simulink model "Diode"  (R2020a)
settings: Solver=VariableStepAuto  StartTime=0.0  StopTime=10.0  RelTol=1e-3
model workspace (MAT data in the model file):
  Eg = Simulink.Parameter
  Eg.Value = 1.23
  Eg.DataType = 'auto'
  Eg.Dimensions = [1 1]
  Is = Simulink.Parameter
  Is.Value = 1.3e-09
  Is.DataType = 'auto'
  Is.Dimensions = [1 1]
  k = Simulink.Parameter
  k.Value = 1.38e-23
  k.DataType = 'auto'
  k.Dimensions = [1 1]
  n = Simulink.Parameter
  n.Value = 2
  n.DataType = 'auto'
  n.Dimensions = [1 1]
  q = Simulink.Parameter
  q.Value = 1.6e-19
  q.DataType = 'auto'
  q.Dimensions = [1 1]
settings Model: Creator=Shivam  LastModifiedBy=Shivam

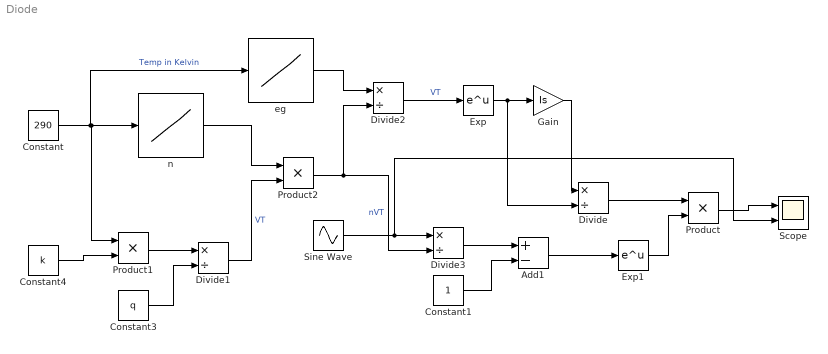
== system Diode ==
  Add1 : Sum  Inputs=+-
  Constant : Constant  Value=290
  Constant1 : Constant
  Constant3 : Constant  Value=q
  Constant4 : Constant  Value=k
  Divide{,1..3} (4 alike) : Product  Inputs=*/
  Exp : Math  SaturateOnIntegerOverflow=on
  Exp1 : Math  SaturateOnIntegerOverflow=on
  Gain : Gain  Gain=Is
  Product : Product
  Product1 : Product
  Product2 : Product
  Scope : Scope  NumInputPorts=2
  Sine Wave : Sin  Amplitude=0.5  SampleTime=0
  eg : Lookup_n-D  NumberOfTableDimensions=1  BreakpointsForDimension1=|  Table=|  InternalRulePriority=Speed  RndMeth=Simplest  InputSameDT=on
      BreakpointsForDimension1=|
      | [150
      | 160
      | 170
      | 180
      | 190
      | 200
      | 210
      | 220
      | 230
      | 240
      | 250
      | 260
      | 270
      | 280
      | 290
      | 300
      | ]
      Table=|
      | [0.39
      | 0.42
      | 0.45
      | 0.48
      | 0.5
      | 0.54
      | 0.56
      | 0.61
      | 0.64
      | 0.66
      | 0.69
      | 0.73
      | 0.75
      | 0.79
      | 0.81
      | 0.83
      | ]
  n : Lookup_n-D  NumberOfTableDimensions=1  BreakpointsForDimension1=|  Table=|  InternalRulePriority=Speed  RndMeth=Simplest  InputSameDT=on
      BreakpointsForDimension1=|
      | [150
      | 160
      | 170
      | 180
      | 190
      | 200
      | 210
      | 220
      | 230
      | 240
      | 250
      | 260
      | 270
      | 280
      | 290
      | 300]
      Table=|
      | [6.95
      | 6.49
      | 6.06
      | 5.66
      | 5.24
      | 5.05
      | 4.46
      | 4.05
      | 3.57
      | 3.21
      | 2.89
      | 2.68
      | 2.65
      | 2.6
      | 2.27
      | 2.04
      | ]
  wires:
  Constant/1 -> eg/1, Product1/1, n/1  "Temp in Kelvin"
  n/1 -> Product2/1
  Constant4/1 -> Product1/2
  Product1/1 -> Divide1/1
  Constant3/1 -> Divide1/2
  Divide1/1 -> Product2/2  "VT"
  Product2/1 -> Divide3/2, Divide2/2  "nVT"
  eg/1 -> Divide2/1
  Divide2/1 -> Exp/1  "VT"
  Exp/1 -> Divide/2, Gain/1
  Gain/1 -> Divide/1
  Sine Wave/1 -> Scope/2, Divide3/1
  Divide3/1 -> Add1/1
  Constant1/1 -> Add1/2
  Add1/1 -> Exp1/1
  Divide/1 -> Product/1
  Exp1/1 -> Product/2
  Product/1 -> Scope/1
